simulink library "roblocks"  (Simulink 7.1)
values from neighbouring files (symbols this model uses):
  q = jtraj(qz, qr, t)    [rtandemo.m]    (also in rtjademo.m = [0.1 0.75 -2.25 0 .75 0]; rttgdemo.m)
undefined symbols (not defined in the file or in its folder): eul2tr, fkine, jacob0, jacobn, qd, qdd, rne, robot, rpy2tr, tr2diff, tr2eul, tr2rpy, transl
libraries: simulink3 x2
settings Model: Creator=pic  LastModifiedBy=pic  ExtModeAutoUpdateStatusClock=off

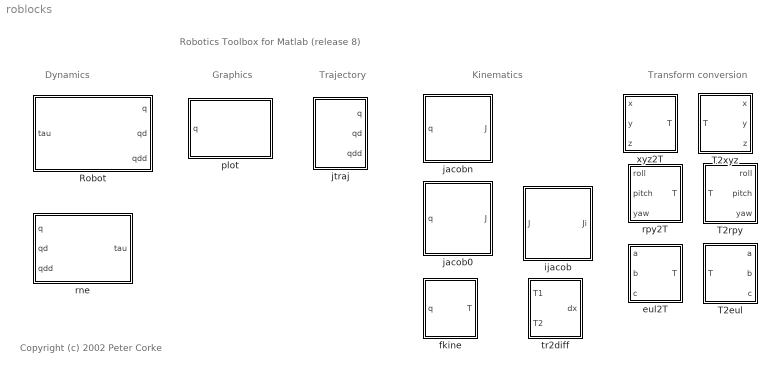
== system roblocks ==
  note: Robotics Toolbox for Matlab (release 8)
  note: Copyright (c) 2002 Peter Corke
  note: Dynamics
  note: Graphics
  note: Kinematics
  note: Transform conversion
  note: Trajectory
  Robot : Subsystem  mask{robot=robot, q0=[0 0 0 0 0 0]}
      mask prompts: robot "Robot object"; q0 "Initial state"
      mask help: Rigid-body dynamic model of robot.
      mask init:
      | n = robot.n;
      | name = robot.name;
      mask Help: Simulates the forward (direct) rigid-body dynamics of the robot described by the given robot object.
      mask Display:
      | port_label('input', 1, 'tau')
      | port_label('output', 1, 'q')
      | port_label('output', 2, 'qd')
      | port_label('output', 3, 'qdd')
      | text(0.1, 0.9,  name, 'horizontalAlignment', 'left')
  T2eul : Subsystem
      mask Description: Convert transform to Euler angles.
  T2rpy : Subsystem
      mask Description: Convert transform to roll/pitch/yaw angles.
  T2xyz : Subsystem
      mask Description: Convert transform to xyz scalars
  eul2T : Subsystem
      mask Description: Convert Euler angles to transform.
  fkine : Subsystem  mask{robot=robot}
      mask prompts: robot "Robot object"
      mask help: Robot forward kinematics.
      mask Help: Compute homogeneous transform for robot end-effector given joint angles.
      mask Display:
      | port_label('input', 1, 'q')
      | port_label('output', 1, 'T')
      | text(0.9, 0.9, robot.name,  'horizontalAlignment', 'right')
  ijacob : Subsystem
      mask Description:
      | Robot inverse Jacobian for world coordinates.
      | 
      | Only valid for square jacobians (ie/ 6DOF robots)
      mask Display:
      | text(0.4, 0.7, 'J', 'verticalAlignment', 'top', 'horizontalAlignment', 'left')
      | text(0.65, 0.65, '-1', 'verticalAlignment', 'bottom', 'horizontalAlignment', 'right')
      | port_label('input', 1, 'J');
      | port_label('output', 1, 'Ji')
  "jacob0 " : Subsystem  mask{robot=robot}
      mask prompts: robot "Robot object"
      mask help: Robot Jacobian for end-effector coordinates
      mask init:
      | n=robot.n;
      mask Display:
      | text(0.4, 0.7, 'J', 'verticalAlignment', 'top', 'horizontalAlignment', 'left')
      | text(0.4, 0.7, '0', 'verticalAlignment', 'bottom', 'horizontalAlignment', 'right')
      | text(0.5, 0.2, robot.name,  'horizontalAlignment', 'center')
      | port_label('input', 1, 'q')
      | port_label('output', 1, 'J')
  jacobn : Subsystem  mask{robot=robot}
      mask prompts: robot "Robot object"
      mask help: Robot Jacobian for end-effector coordinates
      mask init:
      | n=robot.n;
      mask Display:
      | text(0.5, 0.4, 'J', 'verticalAlignment', 'top', 'horizontalAlignment', 'left')
      | text(0.5, 0.4, 'n', 'verticalAlignment', 'bottom', 'horizontalAlignment', 'right')
      | text(0.9, 0.9, robot.name,  'horizontalAlignment', 'right')
      | port_label('input', 1, 'q')
      | port_label('output', 1, 'J')
  jtraj : Subsystem  mask{q0=[0 0 0 0 0 0], qf=[pi/4 pi/2 -pi/2 0 0 0], tmax=10}
      mask help: Joint interpolated trajectory.
      mask init:
      | n = length(q0);
      | if length(q0) ~= length(qf) ,
      |  error('q0 and qf must be same length')
      | end
      | t=[0:100]'/100*tmax;
      | [q,qd,qdd] = jtraj(q0, qf, t);
      mask Help:
      | Generate quintic polynomial to move from initial to final joint angles as specified.  Initial and final velocity are assumed to be zero.
      | 
      | Outputs joint angles as well as joint angle rates.
      mask Display:
      | port_label('output', 1, 'q')
      | port_label('output', 2, 'qd')
      | port_label('output', 3, 'qdd')
  plot : Subsystem  mask{robot=robot}
      mask prompts: robot "Name of robot"
      mask help: Graphical robot display.
      mask init:
      | plot(robot,zeros(1,robot.n));
      | rname = robot.name;
      | fprintf('**robot name is %s\n', rname);
      mask Help: This block graphically displays the named robot
      mask Display: text(0.5, 0.5,  rname, 'horizontalAlignment', 'center')
  rne : Subsystem  mask{robot=robot, grav=[0 0 9.81]}
      mask prompts: robot "Robot object"; grav "Gravity"
      mask help: Rigid-body inverse dynamics.
      mask init:
      | n=robot.n;
      mask Help: Given a robot dynamic model and joint angle, rate and acceleration determine the required joint torque.  Useful for computed and inverse torque control schemes.
      mask Display:
      | port_label('output', 1, 'tau')
      | port_label('input', 1, 'q')
      | port_label('input', 2, 'qd')
      | port_label('input', 3, 'qdd')
      | text(0.9, 0.9,  robot.name, 'horizontalAlignment', 'right')
  rpy2T : Subsystem
      mask Description: Convert roll/pitch/yaw angles to transform.
  tr2diff : Subsystem  mask{robot=robot}
      mask prompts: robot "Robot object"
      mask help: Robot forward kinematics.
      mask Help: Compute homogeneous transform for robot end-effector given joint angles.
      mask Display:
      | port_label('input', 1, 'T1')
      | port_label('input', 2, 'T2')
      | port_label('output', 1, 'dx')
  xyz2T : Subsystem
      mask Description: Convert xyz scalars to transform.

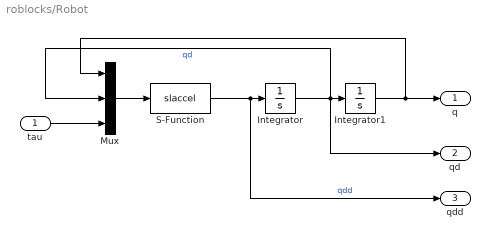
== system roblocks/Robot ==
  tau : Inport  OutDataType=sfix(16)  OutScaling=2^0
  Integrator : Integrator
  Integrator1 : Integrator
  Mux : Mux  Inputs=3
  S-Function : S-Function  FunctionName=slaccel  Parameters=robot  EnableBusSupport=off
  q : Outport
  qd : Outport  Port=2
  qdd : Outport  Port=3
  wires:
  S-Function/1 -> qdd/1, Integrator/1  "qdd"
  Mux/1 -> S-Function/1
  Integrator/1 -> qd/1, Integrator1/1, Mux/2  "qd"
  tau/1 -> Mux/3
  Integrator1/1 -> q/1, Mux/1

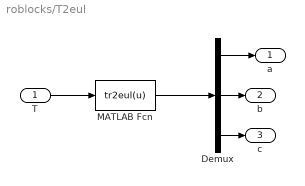
== system roblocks/T2eul ==
  T : Inport
  Demux : Demux  Outputs=3
  MATLAB Fcn : MATLABFcn  MATLABFcn=tr2eul(u)  OutputDimensions=3
  a : Outport
  b : Outport  Port=2
  c : Outport  Port=3
  wires:
  Demux/3 -> c/1
  Demux/2 -> b/1
  Demux/1 -> a/1
  MATLAB Fcn/1 -> Demux/1
  T/1 -> MATLAB Fcn/1

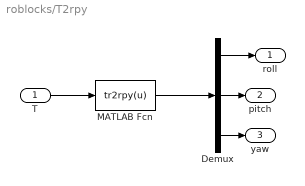
== system roblocks/T2rpy ==
  T : Inport
  Demux : Demux  Outputs=3
  MATLAB Fcn : MATLABFcn  MATLABFcn=tr2rpy(u)  OutputDimensions=3
  roll : Outport
  pitch : Outport  Port=2
  yaw : Outport  Port=3
  wires:
  Demux/3 -> yaw/1
  Demux/2 -> pitch/1
  Demux/1 -> roll/1
  MATLAB Fcn/1 -> Demux/1
  T/1 -> MATLAB Fcn/1

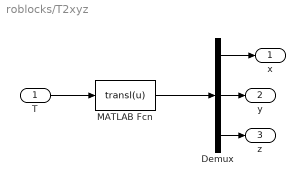
== system roblocks/T2xyz ==
  T : Inport
  Demux : Demux  Outputs=3
  MATLAB Fcn : MATLABFcn  MATLABFcn=transl(u)  OutputDimensions=3
  x : Outport
  y : Outport  Port=2
  z : Outport  Port=3
  wires:
  T/1 -> MATLAB Fcn/1
  MATLAB Fcn/1 -> Demux/1
  Demux/1 -> x/1
  Demux/2 -> y/1
  Demux/3 -> z/1

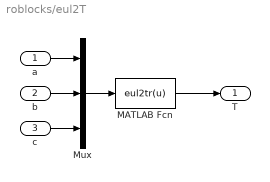
== system roblocks/eul2T ==
  a : Inport
  b : Inport  Port=2
  c : Inport  Port=3
  MATLAB Fcn : MATLABFcn  MATLABFcn=eul2tr(u)  OutputDimensions=[4 4]  Output1D=off
  Mux : Mux  Inputs=3
  T : Outport
  wires:
  c/1 -> Mux/3
  MATLAB Fcn/1 -> T/1
  Mux/1 -> MATLAB Fcn/1
  a/1 -> Mux/1
  b/1 -> Mux/2

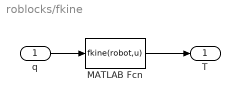
== system roblocks/fkine ==
  q : Inport
  MATLAB Fcn : MATLABFcn  MATLABFcn=fkine(robot,u)  OutputDimensions=[4 4]  Output1D=off
  T : Outport
  wires:
  q/1 -> MATLAB Fcn/1
  MATLAB Fcn/1 -> T/1

== system roblocks/ijacob ==
  J : Inport
  inverse jacobian : MATLABFcn  MATLABFcn=inv(u)  Output1D=off
  Ji : Outport
  wires:
  inverse jacobian/1 -> Ji/1
  J/1 -> inverse jacobian/1

== system roblocks/jacob0  ==
  q : Inport
  MATLAB Fcn : MATLABFcn  MATLABFcn=jacob0(robot,u)  OutputDimensions=[6 n]  Output1D=off
  J : Outport
  wires:
  MATLAB Fcn/1 -> J/1
  q/1 -> MATLAB Fcn/1

== system roblocks/jacobn ==
  q : Inport
  MATLAB Fcn : MATLABFcn  MATLABFcn=jacobn(robot,u)  OutputDimensions=[6 n]  Output1D=off
  J : Outport
  wires:
  MATLAB Fcn/1 -> J/1
  q/1 -> MATLAB Fcn/1

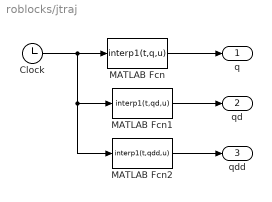
== system roblocks/jtraj ==
  Clock : Clock
      settings: Decimation=10
  MATLAB Fcn : MATLABFcn  MATLABFcn=interp1(t,q,u)  OutputDimensions=n
  MATLAB Fcn1 : MATLABFcn  MATLABFcn=interp1(t,qd,u)  OutputDimensions=n
  MATLAB Fcn2 : MATLABFcn  MATLABFcn=interp1(t,qdd,u)  OutputDimensions=n
  q : Outport
  qd : Outport  Port=2
  qdd : Outport  Port=3
  wires:
  MATLAB Fcn/1 -> q/1
  MATLAB Fcn1/1 -> qd/1
  Clock/1 -> MATLAB Fcn/1, MATLAB Fcn1/1, MATLAB Fcn2/1
  MATLAB Fcn2/1 -> qdd/1

== system roblocks/plot ==
  q : Inport  OutDataType=sfix(16)  OutScaling=2^0
  S-Function : S-Function  FunctionName=slplotbot  Parameters=robot  EnableBusSupport=off
  wires:
  q/1 -> S-Function/1

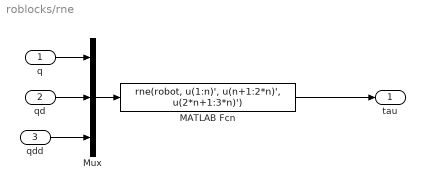
== system roblocks/rne ==
  q : Inport
  qd : Inport  Port=2
  qdd : Inport  Port=3
  MATLAB Fcn : MATLABFcn  MATLABFcn=rne(robot, u(1:n)', u(n+1:2*n)', u(2*n+1:3*n)')  OutputDimensions=n
  Mux : Mux  Inputs=3
  tau : Outport
  wires:
  Mux/1 -> MATLAB Fcn/1
  q/1 -> Mux/1
  qd/1 -> Mux/2
  qdd/1 -> Mux/3
  MATLAB Fcn/1 -> tau/1

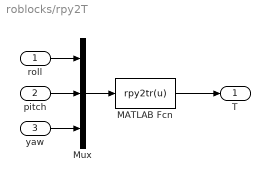
== system roblocks/rpy2T ==
  roll : Inport
  pitch : Inport  Port=2
  yaw : Inport  Port=3
  MATLAB Fcn : MATLABFcn  MATLABFcn=rpy2tr(u)  OutputDimensions=[4 4]  Output1D=off
  Mux : Mux  Inputs=3
  T : Outport
  wires:
  yaw/1 -> Mux/3
  MATLAB Fcn/1 -> T/1
  Mux/1 -> MATLAB Fcn/1
  roll/1 -> Mux/1
  pitch/1 -> Mux/2

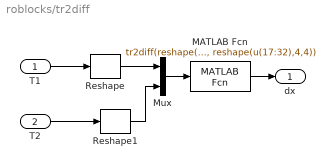
== system roblocks/tr2diff ==
  T1 : Inport
  T2 : Inport  Port=2
  MATLAB Fcn : MATLABFcn  MATLABFcn=tr2diff(reshape(u(1:16),4,4), reshape(u(17:32),4,4))  OutputDimensions=6
  Mux : Mux  Inputs=2
  Reshape : simulink3/Signals & Systems/Reshape  OutputDimensionality=1-D array  OutputDimensions=[1,1]
  Reshape1 : simulink3/Signals & Systems/Reshape  OutputDimensionality=1-D array  OutputDimensions=[1,1]
  dx : Outport
  wires:
  MATLAB Fcn/1 -> dx/1
  T1/1 -> Reshape/1
  T2/1 -> Reshape1/1
  Mux/1 -> MATLAB Fcn/1
  Reshape/1 -> Mux/1
  Reshape1/1 -> Mux/2

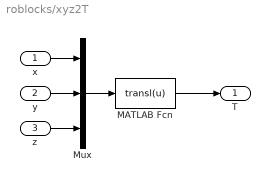
== system roblocks/xyz2T ==
  x : Inport
  y : Inport  Port=2
  z : Inport  Port=3
  MATLAB Fcn : MATLABFcn  MATLABFcn=transl(u)  OutputDimensions=[4 4]  Output1D=off
  Mux : Mux  Inputs=3
  T : Outport
  wires:
  y/1 -> Mux/2
  x/1 -> Mux/1
  Mux/1 -> MATLAB Fcn/1
  MATLAB Fcn/1 -> T/1
  z/1 -> Mux/3
